simulink model "Simulatore_digitale_2"  (Simulink 8.0)
settings: Solver=ode3  StartTime=0.0  StopTime=stop_t  FixedStep=Ts  MaxStep=Ts/10  MinStep=Ts/100  RelTol=1e-3
values from neighbouring files (symbols this model uses):
  a_da = 0    [CA_GIUSE.m]    (also in Script.m)
  a_dp = 2e-2    (= 0.02)    [CA_GIUSE.m]    (also in Script.m = 0)
  a_ds = 0e-1    (= 0)    [CA_GIUSE.m]    (also in Script.m)
  aph = 0.05    [CA_GIUSE.m]    (also in Script.m)
  Da_c = 0e-3    (= 0)    [CA_GIUSE.m]    (also in Script.m)
  Da_r = 00e-1    (= 0)    [CA_GIUSE.m]    (also in Script.m)
  Dp_c = 00e-3    (= 0)    [CA_GIUSE.m]    (also in Script.m)
  Dp_r = 00e-1    (= 0)    [CA_GIUSE.m]    (also in Script.m)
  Ds_c = 00e-3    (= 0)    [CA_GIUSE.m]    (also in Script.m)
  Ds_r = 00e-1    (= 0)    [CA_GIUSE.m]    (also in Script.m)
  Ga = 0e-3    (= 0)    [CA_GIUSE.m]    (also in Script.m)
  Gdp = 0    [CA_GIUSE.m]    (also in Script.m = 1)
  Gf = 1/(Kd*Gs)    [CA_GIUSE.m]    (also in Script.m)
  Gr = 0e0    (= 0)    [CA_GIUSE.m]    (also in Script.m = 1)
  Gs = 0e-0    (= 0)    [CA_GIUSE.m]    (also in Script.m)
  Kd = 0    [CA_GIUSE.m]    (also in Script.m)
  over = 0.1    [CA_GIUSE.m]    (also in Script.m = 0)
  Pulse_da = 0    [CA_GIUSE.m]    (also in Script.m)
  Pulse_dp = 0e-3    (= 0)    [CA_GIUSE.m]    (also in Script.m)
  Pulse_ds = 0    [CA_GIUSE.m]    (also in Script.m)
  R_0 = 1    [CA_GIUSE.m]    (also in Script.m)
  Ts = 0.1/(Wceff); [Gcz,Lz]=TDmode(Ts,Glp,Gc,Ga,Gp,Gs,Gf)    [CA_GIUSE.m]    (also in Script.m)
undefined symbols (not defined in the file or in its folder): den_Gcz, den_Gp, num_Gcz, num_Gp
libraries: simulink x4
settings Model: Creator=Sandro  LastModifiedBy=S156757
settings DataIOCC: SignalLoggingSaveFormat=ModelDataLogs
settings DebuggingCC: FcnCallInpInsideContextMsg=UseLocalSettings
settings GRTTargetCC: CombineOutputUpdateFcns=off  GRTInterface=on

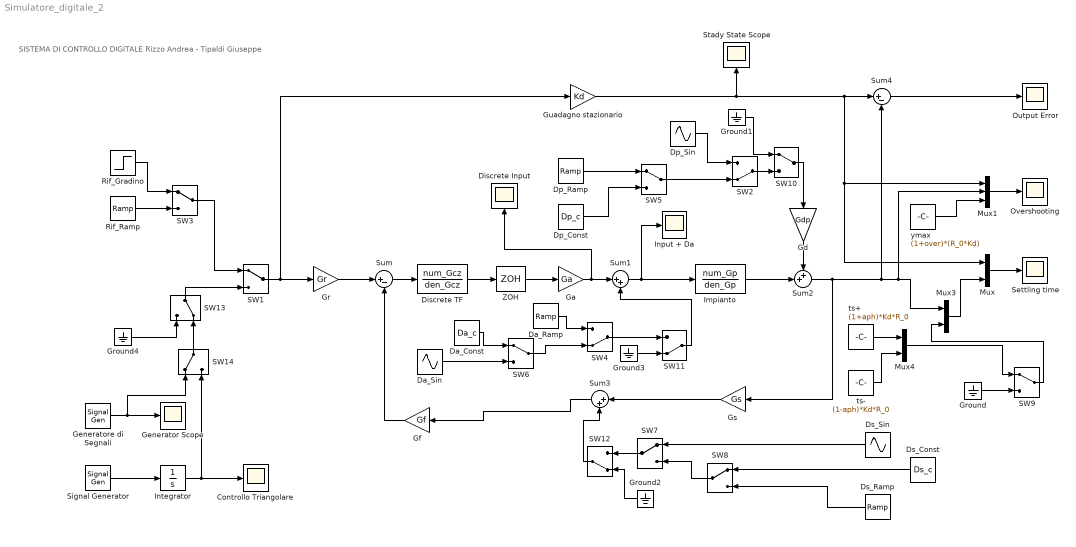
== system Simulatore_digitale_2 ==
  note: SISTEMA DI CONTROLLO DIGITALE
      | Rizzo Andrea - Tipaldi Giuseppe
  Controllo Triangolare : Scope
      settings: SaveName=ScopeData3
  Da_Const : Constant  Value=Da_c
  Da_Ramp : simulink/Sources/Ramp  slope=Da_r  start=0  X0=0
  Da_Sin : Sin  Amplitude=a_da  Frequency=Pulse_da  SampleTime=0
  Discrete Input : Scope
      settings: TimeRange=7.62942779291553  YMin=0.9536585365853658  YMax=1.036585365853659  SaveName=ScopeData4
  Discrete TF : DiscreteTransferFcn  Numerator=num_Gcz  Denominator=den_Gcz  SampleTime=Ts
  Dp_Const : Constant  Value=Dp_c
  Dp_Ramp : simulink/Sources/Ramp  slope=Dp_r  start=0  X0=0
  Dp_Sin : Sin  Amplitude=a_dp  Frequency=Pulse_dp  SampleTime=0
  Ds_Const : Constant  Value=Ds_c
  Ds_Ramp : simulink/Sources/Ramp  slope=Ds_r  start=0  X0=0
  Ds_Sin : Sin  Amplitude=a_ds  Frequency=Pulse_ds  SampleTime=0
  Ga : Gain  Gain=Ga
  Gd : Gain  Gain=Gdp
  Generator Scope : Scope
      settings: TimeRange=0.002216033935546875  YMin=2.1909418072197  YMax=2.191153294711311  SaveName=ScopeData6
  Generatore di Segnali : SignalGenerator  WaveForm=square  Amplitude=0.5  Frequency=0.25
  Gf : Gain  Gain=Gf
  Gr : Gain  Gain=Gr
  Ground{,1..4} (5 alike) : Ground
  Gs : Gain  Gain=Gs
  Guadagno stazionario : Gain  Gain=Kd
  Impianto : TransferFcn  Numerator=num_Gp  Denominator=den_Gp
  Input + Da : Scope
      settings: TimeRange=7.62942779291553  YMin=0.9536585365853658  YMax=1.036585365853659
  Integrator : Integrator  InitialCondition=0.5
  Mux : Mux  Inputs=2
  Mux1 : Mux  Inputs=3
  Mux3 : Mux  Inputs=2
  Mux4 : Mux  Inputs=2
  Output Error : Scope
      settings: TimeRange=0.2443152625475258  YMin=-0.0007  YMax=0.0007  SaveName=ScopeData2
  Overshooting : Scope
      settings: TimeRange=2.720306513409963  YMin=1.082326936558659  YMax=1.08232813122829  SaveName=ScopeData5
  Rif_Gradino : Step  Time=0  SampleTime=0
  Rif_Ramp : simulink/Sources/Ramp  slope=R_0  start=0  X0=0
  SW{1,3,5..10,14} (9 alike) : ManualSwitch
  SW{2,4,11..13} (5 alike) : ManualSwitch  CurrentSetting=0
  Settling time : Scope
      settings: TimeRange=10  YMin=0  YMax=3.5
  Signal Generator : SignalGenerator  WaveForm=square  Amplitude=0.5  Frequency=0.25
  Stady State Scope : Scope
      settings: TimeRange=7.62942779291553  YMin=0.9536585365853658  YMax=1.036585365853659  SaveName=ScopeData7
  Sum : Sum  Inputs=|+-
  Sum1 : Sum  Inputs=|++
  Sum2 : Sum  Inputs=++|
  Sum3 : Sum  Inputs=|++
  Sum4 : Sum  Inputs=|+-
  ZOH : ZeroOrderHold  SampleTime=Ts
  ts+ : Constant  Value=(1+aph)*Kd*R_0
  ts- : Constant  Value=(1-aph)*Kd*R_0
  ymax : Constant  Value=(1+over)*(R_0*Kd)
  wires:
  Sum/1 -> Discrete TF/1
  Sum1/1 -> Impianto/1, Input + Da/1
  Sum2/1 -> Gs/1, Sum4/2, Mux3/1, Mux1/2
  Ga/1 -> Sum1/1, Discrete Input/1
  Discrete TF/1 -> ZOH/1
  ZOH/1 -> Ga/1
  Guadagno stazionario/1 -> Sum4/1, Mux/1, Mux1/1, Stady State Scope/1
  Mux/1 -> Settling time/1
  Signal Generator/1 -> Integrator/1
  Impianto/1 -> Sum2/2
  Gd/1 -> Sum2/1
  Gs/1 -> Sum3/1
  Gf/1 -> Sum/2
  Gr/1 -> Sum/1
  SW5/1 -> SW2/2
  SW6/1 -> SW4/2
  Dp_Const/1 -> SW5/2
  Dp_Sin/1 -> SW2/1
  Dp_Ramp/1 -> SW5/1
  Da_Sin/1 -> SW6/2
  Da_Const/1 -> SW6/1
  Da_Ramp/1 -> SW4/1
  Rif_Ramp/1 -> SW3/2
  Rif_Gradino/1 -> SW3/1
  SW8/1 -> SW7/2
  Ds_Sin/1 -> SW7/1
  Ds_Const/1 -> SW8/1
  Ds_Ramp/1 -> SW8/2
  Sum4/1 -> Output Error/1
  ts-/1 -> Mux4/2
  ts+/1 -> Mux4/1
  Mux4/1 -> SW9/1
  SW9/1 -> Mux3/2
  Ground/1 -> SW9/2
  Mux1/1 -> Overshooting/1
  SW2/1 -> SW10/2
  SW10/1 -> Gd/1
  Ground1/1 -> SW10/1
  SW7/1 -> SW12/1
  SW12/1 -> Sum3/2
  Ground2/1 -> SW12/2
  SW4/1 -> SW11/1
  Ground3/1 -> SW11/2
  SW11/1 -> Sum1/2
  Generatore di Segnali/1 -> Generator Scope/1, SW14/1
  Mux3/1 -> Mux/2
  Integrator/1 -> Controllo Triangolare/1, SW14/2
  SW1/1 -> Gr/1, Guadagno stazionario/1
  ymax/1 -> Mux1/3
  SW13/1 -> SW1/2
  SW3/1 -> SW1/1
  Ground4/1 -> SW13/1
  SW14/1 -> SW13/2
  Sum3/1 -> Gf/1
